simulink model "COMP_SYS_earth_checkered"  (R2026b)
(part 3 of 19)

  T_A21/LConn1 -- T_B20/RConn1
  T_A65/LConn1 -- T_B57/RConn1
  T_A13/RConn1 -- T_B13/LConn1
  T_A14/LConn1 -- T_B13/RConn1
  T_A18/LConn1 -- T_B31/RConn1
  T_B11/RConn1 -- T_A12/LConn1
  T_A61/RConn1 -- T_B61/LConn1
  T_A11/RConn1 -- T_B11/LConn1
  T_A9/RConn1 -- T_B9/LConn1
  T_A1/RConn1 -- T_B1/LConn1
  T_A95/RConn1 -- T_B95/LConn1
  T_A59/LConn1 -- T_B58/RConn1
  T_A11/LConn1 -- T_B10/RConn1
  T_A2/RConn1 -- T_B2/LConn1
  T_A3/RConn1 -- T_B3/LConn1
  T_A10/LConn1 -- T_B9/RConn1
  T_A85/RConn1 -- T_B85/LConn1
  T_A74/RConn2 -- T_B89/LConn3
  T_A1/LConn1 -- T_B/RConn1
  T_B71/RConn1 -- T_A82/LConn1
  T_B72/RConn2 -- T_A74/LConn3
  T_A73/RConn1 -- T_B73/LConn1
  T_B19/RConn1 -- T_A20/LConn1
  T_A68/RConn1 -- T_B68/LConn1
  T_A77/LConn1 -- T_B76/RConn1
  T_A31/RConn1 -- T_B31/LConn1
  T_B30/RConn2 -- T_A32/LConn3
  T_A17/RConn1 -- T_B17/LConn1
  T_A56/RConn1 -- T_B56/LConn1
  T_A18/RConn1 -- T_B18/LConn1
  T_A58/RConn1 -- T_B58/LConn1
  T_A9/LConn1 -- T_B8/RConn1
  T_A40/RConn1 -- T_B40/LConn1
  T_A43/RConn1 -- T_B43/LConn1
  T_A3/LConn1 -- T_B2/RConn1
  T_A32/RConn1 -- T_B32/LConn1
  T_A32/RConn2 -- T_B46/LConn3
  T_A35/RConn1 -- T_B35/LConn1
  T_A2/LConn1 -- T_B1/RConn1
  T_B8/RConn2 -- T_A16/LConn3
  T_A76/LConn1 -- T_B90/RConn1
  T_B46/RConn2 -- T_A48/LConn3
  T_B35/RConn1 -- T_A36/LConn1
  T_A16/RConn1 -- T_B16/LConn1
  T_A77/RConn1 -- T_B77/LConn1
  T_A33/LConn1 -- T_B32/RConn1
  T_A95/LConn1 -- T_B94/RConn1
  T_A26/RConn1 -- T_B26/LConn1
  T_A68/LConn1 -- T_B67/RConn1
  T_A24/LConn1 -- T_B17/RConn1
  T_A21/RConn1 -- T_B21/LConn1
  T_A57/RConn1 -- T_B57/LConn1
  T_A27/LConn1 -- T_B26/RConn1
  T_A/RConn1 -- T_B/LConn1
  T_A38/LConn1 -- T_B37/RConn1
  T_A60/LConn1 -- T_B49/RConn1
  T_A25/RConn1 -- T_B25/LConn1
  T_A/RConn2 -- T_B8/LConn3
  T_A62/RConn1 -- T_B62/LConn1
  T_A43/LConn1 -- T_B42/RConn1
  T_A65/RConn1 -- T_B65/LConn1
  T_A35/LConn1 -- T_B34/RConn1
  T_A76/RConn1 -- T_B76/LConn1
  T_A19/LConn1 -- T_B18/RConn1
  T_A4/RConn1 -- T_B4/LConn1
  T_A20/RConn1 -- T_B20/LConn1
  T_A36/RConn1 -- T_B36/LConn1
  T_A47/LConn1 -- T_B46/RConn1
  T_A41/RConn1 -- T_B41/LConn1
  T_A42/RConn1 -- T_B42/LConn1
  T_B41/RConn1 -- T_A42/LConn1
  T_A37/LConn1 -- T_B36/RConn1
  T_A27/RConn1 -- T_B27/LConn1
  T_A17/LConn1 -- T_B16/RConn1
  T_B3/RConn1 -- T_A4/LConn1
  T_A54/LConn1 -- T_B53/RConn1
  T_A34/LConn1 -- T_B47/RConn1
  T_A5/LConn1 -- T_B4/RConn1
  T_A19/RConn1 -- T_B19/LConn1
  T_A22/LConn1 -- T_B21/RConn1
  T_A24/RConn1 -- T_B24/LConn1
  T_A5/RConn1 -- T_B5/LConn1
  T_A37/RConn1 -- T_B37/LConn1
  T_A16/RConn2 -- T_B30/LConn3
  FLOOR_SW_CORNER/RConn1 -- T_A/LConn4
